simulink model "Optimal_Slip_Estimator_2016a"  (R2016a)
settings: Solver=VariableStepAuto  SolverMode=SingleTasking  StartTime=0.0  StopTime=10.0  RelTol=1e-3
undefined symbols (not defined in the file): DiscIntNeverNeededParam, OSE_Ts, R, reduction
libraries: simulink x2
settings Model: Creator=univ4123  LastModifiedBy=univ4123
settings DebuggingCC: SFUnexpectedBacktrackingDiag=error  SFNoUnconditionalDefaultTransitionDiag=error
settings SFSimCC: SimUseLocalCustomCode=on
settings RTWCC: RTWUseLocalCustomCode=on
settings GRTTargetCC: TargetLangStandard=C99 (ISO)  GeneratePreprocessorConditionals=Use local settings
settings ConfigComp: CovMetricSettings=dwe  CovHtmlReporting=off  CovSaveCumulativeToWorkspaceVar=off  CovSaveSingleToWorkspaceVar=off  CovExternalEMLEnable=on

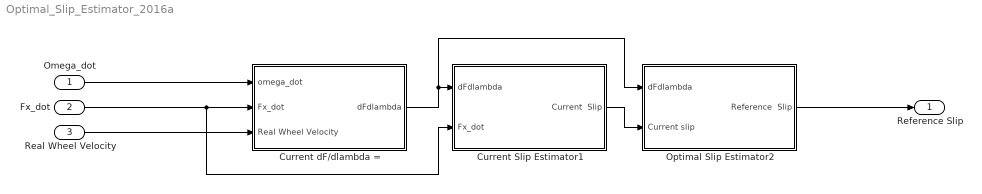
== system Optimal_Slip_Estimator_2016a ==
  Omega_dot : Inport
  Fx_dot : Inport  Port=2
  Real Wheel Velocity : Inport  Port=3
  Current Slip Estimator1 : Subsystem
  Current dF/dlambda = : Subsystem
  Optimal Slip Estimator2 : Subsystem
  Reference Slip : Outport
  wires:
  Omega_dot/1 -> Current dF/dlambda =/1(omega_dot)
  Current dF/dlambda =/1(dFdlambda) -> Optimal Slip Estimator2/1("dFdlambda "), Current Slip Estimator1/1("dFdlambda ")
  Real Wheel Velocity/1 -> Current dF/dlambda =/3(Real Wheel Velocity)
  Fx_dot/1 -> Current Slip Estimator1/2(Fx_dot), Current dF/dlambda =/2(Fx_dot)
  Current Slip Estimator1/1(" Current  Slip") -> Optimal Slip Estimator2/2("Current slip ")
  Optimal Slip Estimator2/1(" Reference  Slip") -> Reference Slip/1

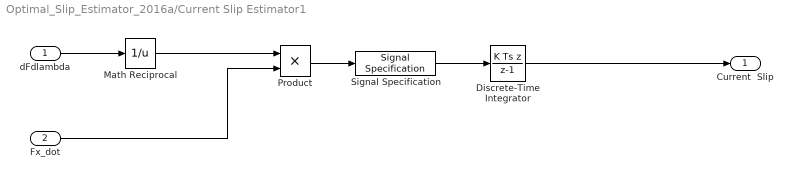
== system Optimal_Slip_Estimator_2016a/Current Slip Estimator1 ==
  "dFdlambda " : Inport
  Fx_dot : Inport  Port=2
  Discrete-Time Integrator : DiscreteIntegrator  IntegratorMethod=Integration: Backward Euler  InitialConditionSetting=State (most efficient)  SampleTime=OSE_Ts  ICPrevOutput=DiscIntNeverNeededParam  ICPrevScaledInput=DiscIntNeverNeededParam
  Math Reciprocal : Math  Operator=reciprocal  SaturateOnIntegerOverflow=on
  Product : Product
  Signal Specification : SignalSpecification  OutDataTypeStr=double
  " Current  Slip" : Outport
  wires:
  "dFdlambda "/1 -> Math Reciprocal/1
  Fx_dot/1 -> Product/2
  Math Reciprocal/1 -> Product/1
  Product/1 -> Signal Specification/1
  Signal Specification/1 -> Discrete-Time Integrator/1
  Discrete-Time Integrator/1 -> " Current  Slip"/1

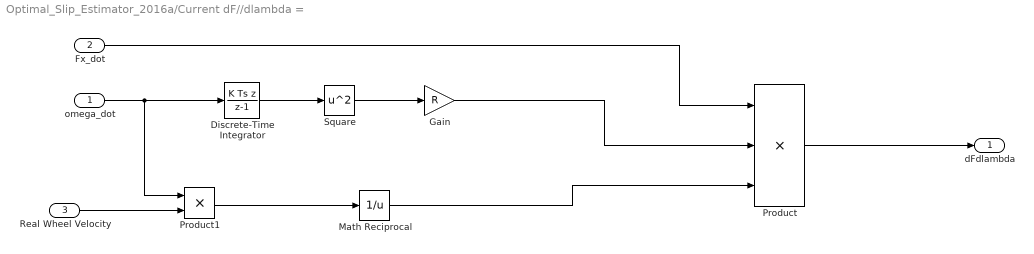
== system Optimal_Slip_Estimator_2016a/Current dF//dlambda = ==
  omega_dot : Inport
  Fx_dot : Inport  Port=2
  Real Wheel Velocity : Inport  Port=3
  Discrete-Time Integrator : DiscreteIntegrator  IntegratorMethod=Integration: Backward Euler  InitialConditionSetting=State (most efficient)  SampleTime=OSE_Ts  ICPrevOutput=DiscIntNeverNeededParam  ICPrevScaledInput=DiscIntNeverNeededParam
  Gain : Gain  Gain=R
  Math Reciprocal : Math  Operator=reciprocal  SaturateOnIntegerOverflow=on
  Product : Product  Inputs=3
  Product1 : Product
  Square : Math  Operator=square  SaturateOnIntegerOverflow=on
  dFdlambda : Outport
  wires:
  omega_dot/1 -> Discrete-Time Integrator/1, Product1/1
  Discrete-Time Integrator/1 -> Square/1
  Square/1 -> Gain/1
  Fx_dot/1 -> Product/1
  Gain/1 -> Product/2
  Real Wheel Velocity/1 -> Product1/2
  Product1/1 -> Math Reciprocal/1
  Math Reciprocal/1 -> Product/3
  Product/1 -> dFdlambda/1

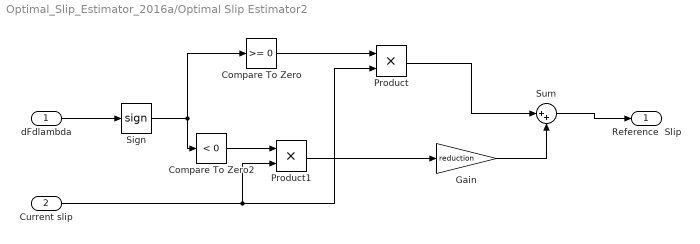
== system Optimal_Slip_Estimator_2016a/Optimal Slip Estimator2 ==
  "dFdlambda " : Inport
  "Current slip " : Inport  Port=2
  Compare To Zero : simulink/Logic and Bit Operations/Compare To Zero  relop=>=  OutDataTypeStr=boolean
  Compare To Zero2 : simulink/Logic and Bit Operations/Compare To Zero  relop=<  OutDataTypeStr=boolean
  Gain : Gain  Gain=reduction
  Product : Product
  Product1 : Product
  Sign : Signum
  Sum : Sum  Inputs=|++
  " Reference  Slip" : Outport
  wires:
  Sign/1 -> Compare To Zero2/1, Compare To Zero/1
  "dFdlambda "/1 -> Sign/1
  Compare To Zero2/1 -> Product1/1
  Gain/1 -> Sum/2
  Product/1 -> Sum/1
  Sum/1 -> " Reference  Slip"/1
  "Current slip "/1 -> Product1/2, Product/2
  Product1/1 -> Gain/1
  Compare To Zero/1 -> Product/1
